simulink model "lineChange"  (R2023b)
settings: Solver=VariableStepAuto  StartTime=0.0  StopTime=10.0  RelTol=1e-3
settings Model: Creator=neham  LastModifiedBy=neham

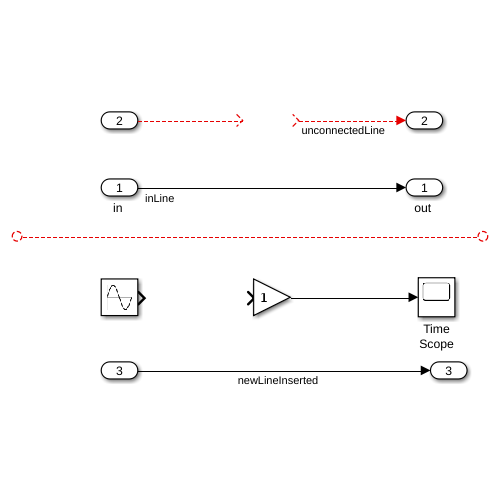
[thumbnail: Simulink's stored preview of the top-level diagram]
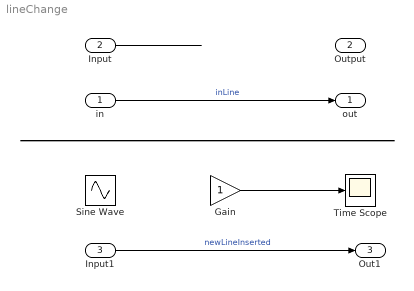
== system lineChange ==
  "in " : Inport
  Input : Inport  Port=2
  Input1 : Inport  Port=3
  Gain : Gain
  Sine Wave : Sin  SampleTime=0
  Time Scope : Scope
  "out " : Outport
  Output : Outport  Port=2
  Out1 : Outport  Port=3
  wires:
  Gain/1 -> Time Scope/1
  "in "/1 -> "out "/1  "inLine"
  Input/1 -> ?
  ? -> Output/1  "unconnectedLine"
  Input1/1 -> Out1/1  "newLineInserted"
  connections:
  ?
